simulink model "popc"  (R2015b)
settings: Solver=FixedStepAuto  StartTime=0.0  StopTime=5  RelTol=1e-3
values from neighbouring files (symbols this model uses):
  b = block.DialogPrm(1).Data    [controller_less.m]    (also in controller_more.m)
  BWall = 0    [Initial_Conditions.m]
  KWall = 10000    [Initial_Conditions.m]
  m = 1    [Initiation.m]
  nWall = block.DialogPrm(6).Data    [Controller1.m]    (also in HapticController.m = block.DialogPrm(3).Data; Initial_Conditions.m = -1; Initiation.m = -1; MoreConservative.m = block.DialogPrm(5).Data)
  x0 = block.DialogPrm(5).Data    [HapticDevice.m]    (also in HumanOperator.m; LessConservative.m = block.DialogPrm(3).Data; MoreConservative.m = block.DialogPrm(3).Data)
  xWall = 0.126    [Initiation.m]    (also in MoreConservative.m = block.DialogPrm(4).Data; Parameters.m = [1 2 3 4 5 6 7 8]*0.0005; VirtualEnvironment.m = block.DialogPrm(3).Data; VirtualEnvironment5.m = block.DialogPrm(4).Data)
undefined symbols (not defined in the file or in its folder): DiscIntNeverNeededParam, Fhand, sigbuilder_block, tWall, x_dot0
libraries: simulink x1
settings Model: Creator=TOSHIBA  LastModifiedBy=TOSHIBA

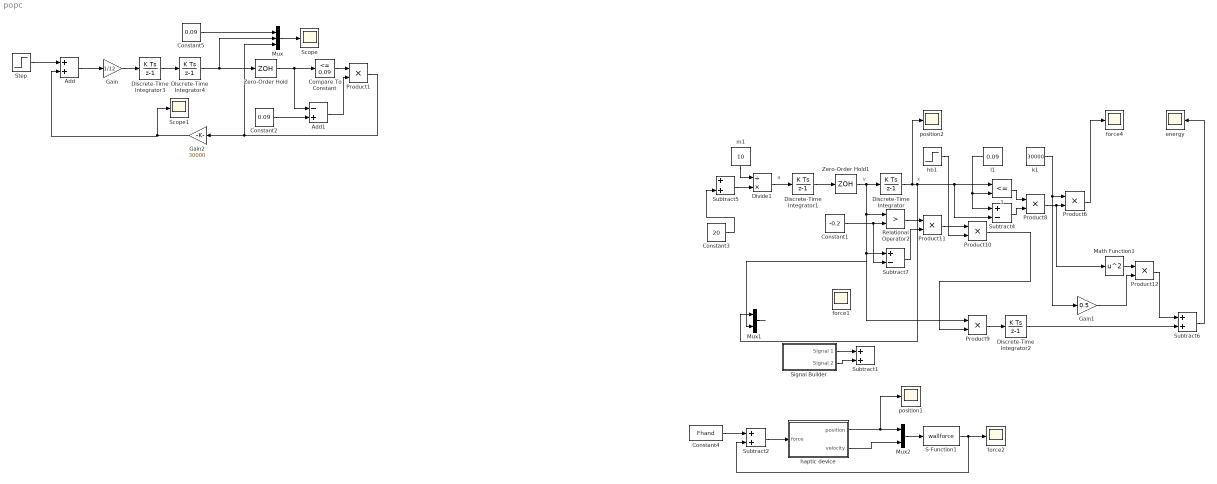
== system popc ==
  note: x
  note: v
  note: a
  " 1" : RelationalOperator  Operator=<=  OutDataTypeStr=boolean
  Add : Sum
  Add1 : Sum  Inputs=-+
  Compare To Constant : simulink/Logic and Bit Operations/Compare To Constant  relop=<=  const=0.09  OutDataTypeStr=boolean
  Constant1 : Constant  Value=-0.2
  Constant2 : Constant  Value=0.09
  Constant3 : Constant  Value=20
  Constant4 : Constant  Value=Fhand
  Constant5 : Constant  Value=0.09
  Discrete-Time Integrator : DiscreteIntegrator  InitialCondition=0.14  InitialConditionSetting=State (most efficient)  SampleTime=0.015  ICPrevOutput=DiscIntNeverNeededParam  ICPrevScaledInput=DiscIntNeverNeededParam
  Discrete-Time Integrator1 : DiscreteIntegrator  InitialConditionSetting=State (most efficient)  SampleTime=0.015  ICPrevOutput=DiscIntNeverNeededParam  ICPrevScaledInput=DiscIntNeverNeededParam
  Discrete-Time Integrator2 : DiscreteIntegrator  InitialConditionSetting=State (most efficient)  SampleTime=0.015  ICPrevOutput=DiscIntNeverNeededParam  ICPrevScaledInput=DiscIntNeverNeededParam
  Discrete-Time Integrator3 : DiscreteIntegrator  InitialConditionSetting=State (most efficient)  SampleTime=0.015  ICPrevOutput=DiscIntNeverNeededParam  ICPrevScaledInput=DiscIntNeverNeededParam
  Discrete-Time Integrator4 : DiscreteIntegrator  InitialCondition=0.14  InitialConditionSetting=State (most efficient)  SampleTime=0.015  ICPrevOutput=DiscIntNeverNeededParam  ICPrevScaledInput=DiscIntNeverNeededParam
  Divide1 : Product  Inputs=/*
  Gain : Gain  Gain=1/12
  Gain1 : Gain  Gain=0.5
  Gain2 : Gain  Gain=30000
  Math Function1 : Math  Operator=square  SaturateOnIntegerOverflow=on
  Mux : Mux  Inputs=3
  Mux1 : Mux  Inputs=2
  Mux2 : Mux  Inputs=2
  Product{1,6,8..12} (7 alike) : Product
  Relational Operator2 : RelationalOperator  Operator=>  OutDataTypeStr=boolean
  S-Function1 : S-Function  FunctionName=wallforce  Parameters=xWall,KWall,BWall,nWall,tWall  SFunctionDeploymentMode=off  EnableBusSupport=off
  Scope : Scope
  Scope1 : Scope
  Signal Builder : Subsystem  Tag=STV Subsys  LoadFcn=sigbuilder_block('load');  StartFcn=sigbuilder_block('start');  StopFcn=sigbuilder_block('stop');  ClipboardFcn=sigbuilder_block('clipboard');  mask(Sigbuilder block){}
      mask help: Simulink:masks:SigbuilderBlock_MD
      mask init:
      | if ~strcmp(get_param(bdroot(gcbh),'SimulationStatus'),'stopped') tuvar = sigbuilder_block('maskInit'); end
      settings: CopyFcn=sigbuilder_block('copy');  DeleteFcn=sigbuilder_block('delete');  ModelCloseFcn=sigbuilder_block('modelClose');  PreSaveFcn=sigbuilder_block('preSave');  PauseFcn=sigbuilder_block('pause');  ContinueFcn=sigbuilder_block('continue');  NameChangeFcn=sigbuilder_block('namechange');  OpenFcn=sigbuilder_block('open',[437.25 153.75 550.5 358.5 ]);  CloseFcn=sigbuilder_block('close');
      mask Display: plot(0, 0, 100, 100,[2, 2, 32, 32, 2], [68, 8, 8, 68, 68],[32, 2], [38, 38], [32, 19, 2],[53, 60, 44], [32, 17, 17, 2],[16, 16, 31, 31]);txt = getActiveGroup(gcbh);text(2, 100, txt,'verticalAlignment', 'top');
  Step : Step  After=-30  SampleTime=0.015
  Subtract{1..2,5..6} (4 alike) : Sum
  Subtract4 : Sum  Inputs=+-
  Subtract7 : Sum  Inputs=+-
  Zero-Order Hold : ZeroOrderHold  SampleTime=0.015
  Zero-Order Hold1 : ZeroOrderHold  SampleTime=0.015
  energy : Scope
  force1 : Scope
  force2 : Scope
  force4 : Scope
  haptic device : Subsystem
  hb1 : Step  After=-100  SampleTime=0.015
  k1 : Constant  Value=30000
  l1 : Constant  Value=0.09
  m1 : Constant  Value=10
  position1 : Scope
  position2 : Scope
  wires:
  Add/1 -> Gain/1
  Gain2/1 -> Add/2, Scope1/1
  Step/1 -> Add/1
  Constant2/1 -> Add1/2
  Compare To Constant/1 -> Product1/1
  Add1/1 -> Product1/2
  Mux/1 -> Scope/1
  Constant5/1 -> Mux/1
  Product1/1 -> Mux/3, Gain2/1
  Zero-Order Hold/1 -> Add1/1, Compare To Constant/1
  Gain/1 -> Discrete-Time Integrator3/1
  Discrete-Time Integrator4/1 -> Mux/2, Zero-Order Hold/1
  k1/1 -> Product6/1, Gain1/1
  Subtract4/1 -> Product8/2
  " 1"/1 -> Product8/1
  Subtract5/1 -> Divide1/2
  Constant1/1 -> Relational Operator2/2, Subtract7/2
  Subtract7/1 -> Product11/2
  Product10/1 -> Product9/2
  Product6/1 -> force4/1
  m1/1 -> Divide1/1
  l1/1 -> " 1"/2, Subtract4/1
  Divide1/1 -> Discrete-Time Integrator1/1
  Math Function1/1 -> Product12/1
  Gain1/1 -> Product12/2
  Relational Operator2/1 -> Product11/1
  Product8/1 -> Math Function1/1, Product6/2
  Product12/1 -> Subtract6/1
  Subtract6/1 -> energy/1
  Product11/1 -> Product10/1
  Discrete-Time Integrator1/1 -> Zero-Order Hold1/1
  Zero-Order Hold1/1 -> Mux1/2, Product9/1, Subtract7/1, Relational Operator2/1, Discrete-Time Integrator/1
  Discrete-Time Integrator/1 -> position2/1, Mux1/1, Subtract4/2, " 1"/1
  Product9/1 -> Discrete-Time Integrator2/1
  Discrete-Time Integrator2/1 -> Subtract6/2
  Discrete-Time Integrator3/1 -> Discrete-Time Integrator4/1
  Signal Builder/1(Signal 1) -> Subtract1/1
  Signal Builder/2(Signal 2) -> Subtract1/2
  hb1/1 -> Product10/2
  Mux1/1 -> ?
  ? -> force1/1, Subtract5/1
  Constant3/1 -> Subtract5/2
  haptic device/1(position) -> position1/1, Mux2/1
  haptic device/2(velocity) -> Mux2/2
  Mux2/1 -> S-Function1/1
  Subtract2/1 -> haptic device/1(force)
  S-Function1/1 -> force2/1, Subtract2/2
  Constant4/1 -> Subtract2/1

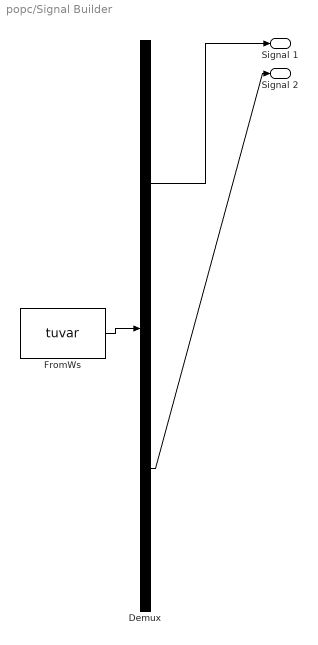
== system popc/Signal Builder ==
  Demux : Demux  Tag=STV Demux  Outputs=2
  FromWs : FromWorkspace  Tag=STV FromWs  VariableName=tuvar  SampleTime=0
      SigBuilderData=|
      | common.afterFinalStr = 'Extrapolate'
      | common.sampleTime = 0
      | dataSet.timeRange = [0 10]
      | dataSet.name = 'Group 1'
      | sbobj.Groups.Name = 'Group 1'
      | sbobj.Groups.Signals(1).Name = 'Signal 1'
      | sbobj.Groups.Signals(1).XData = [0 1 1 1.4 1.4 10]
      | sbobj.Groups.Signals(1).YData = [0 0 -100 -100 0 0]
      | sbobj.Groups.Signals(2).Name = 'Signal 2'
      | sbobj.Groups.Signals(2).XData = [0 1.4 1.4 10]
      | sbobj.Groups.Signals(2).YData = [0 0 -500 -500]
  Signal 1 : Outport  Tag=STV Outport
  Signal 2 : Outport  Tag=STV Outport  Port=2
  wires:
  Demux/1 -> Signal 1/1
  FromWs/1 -> Demux/1
  Demux/2 -> Signal 2/1

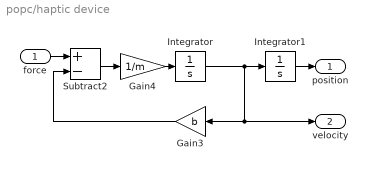
== system popc/haptic device ==
  force : Inport
  Gain3 : Gain  Gain=b
  Gain4 : Gain  Gain=1/m
  Integrator : Integrator  InitialCondition=x_dot0
  Integrator1 : Integrator  InitialCondition=x0
  Subtract2 : Sum  Inputs=+-
  position : Outport
  velocity : Outport  Port=2
  wires:
  force/1 -> Subtract2/1
  Integrator1/1 -> position/1
  Subtract2/1 -> Gain4/1
  Gain4/1 -> Integrator/1
  Gain3/1 -> Subtract2/2
  Integrator/1 -> velocity/1, Gain3/1, Integrator1/1
